simulink model "Coupled_USV_2DOF_SS_tcurve_wPID_FF_curves_2015"  (R2015b)
settings: Solver=VariableStepAuto  StartTime=0.0  StopTime=10  RelTol=1e-3
values from neighbouring files (symbols this model uses):
  breakpoints1 = data(end:-1:1,1)'    [Experimental_Impl.m]    (also in Experimental_Impl_wPlot.m; FEB02_LAKE_TEST.m; FEB14_LAKE_TEST.m; FEB28_LAKE_TEST.m)
  drag_coeff = 16.91    [Experimental_Impl.m]    (also in Experimental_Impl_wPlot.m; FEB02_LAKE_TEST.m = 8.5; FEB02_Post_Processing.m; FEB14_LAKE_TEST.m)
  Kds = .01    (= 0.01)    [FEB02_LAKE_TEST.m]    (also in FEB02_Post_Processing.m = Gain_S(3,i); FEB14_LAKE_TEST.m; FEB28_LAKE_TEST.m = 0; GainIteration_Coup.m = Gain_S(3,i))
  Kdy = Gain(3,i)    [Experimental_Impl.m]    (also in Experimental_Impl_wPlot.m; FEB02_LAKE_TEST.m = 20; FEB02_Post_Processing.m = Gain_Y(3,k); FEB14_LAKE_TEST.m = 20)
  Kis = 7    [FEB02_LAKE_TEST.m]    (also in FEB02_Post_Processing.m = Gain_S(2,i); FEB14_LAKE_TEST.m; FEB28_LAKE_TEST.m = 15; GainIteration_Coup.m = Gain_S(2,i))
  Kiy = Gain(2,i)    [Experimental_Impl.m]    (also in Experimental_Impl_wPlot.m; FEB02_LAKE_TEST.m = 0.01; FEB02_Post_Processing.m = Gain_Y(2,k); FEB14_LAKE_TEST.m = 0.01)
  Kps = 12    [FEB02_LAKE_TEST.m]    (also in FEB02_Post_Processing.m = Gain_S(1,i); FEB14_LAKE_TEST.m; FEB28_LAKE_TEST.m = 40; GainIteration_Coup.m = Gain_S(1,i))
  Kpy = Gain(1,i)    [Experimental_Impl.m]    (also in Experimental_Impl_wPlot.m; FEB02_LAKE_TEST.m = 100; FEB02_Post_Processing.m = Gain_Y(1,k); FEB14_LAKE_TEST.m = 100)
  switch_case = 0    [Experimental_Impl.m]    (also in Experimental_Impl_wPlot.m; FEB02_LAKE_TEST.m = 1; FEB02_Post_Processing.m; FEB14_LAKE_TEST.m)
  table_data = data(end:-1:1,2)'    [Experimental_Impl.m]    (also in Experimental_Impl_wPlot.m; FEB02_LAKE_TEST.m; FEB14_LAKE_TEST.m; FEB28_LAKE_TEST.m)
  vf = 0.0    (= 0)    [Experimental_Impl.m]    (also in Experimental_Impl_wPlot.m; FEB02_LAKE_TEST.m = 1.5; FEB02_Post_Processing.m = 1.25; FEB14_LAKE_TEST.m = 1.5)
  vo = 0.0    (= 0)    [Experimental_Impl.m]    (also in Experimental_Impl_wPlot.m; FEB02_LAKE_TEST.m = 1.25; FEB02_Post_Processing.m = 1.25; FEB14_LAKE_TEST.m = 1.25)
  yf = pi/4    (= 0.785398163397)    [Experimental_Impl.m]    (also in Experimental_Impl_wPlot.m = 0; FEB02_LAKE_TEST.m = 0; FEB02_Post_Processing.m = pi()/4; FEB14_LAKE_TEST.m = 0)
  yo = 0    [Experimental_Impl.m]    (also in Experimental_Impl_wPlot.m; FEB02_LAKE_TEST.m; FEB02_Post_Processing.m; FEB14_LAKE_TEST.m)
libraries: simulink_extras x1
settings Model: Creator=bsb  LastModifiedBy=aschnieders22
settings ConfigComp: CovModelRefEnable=Off

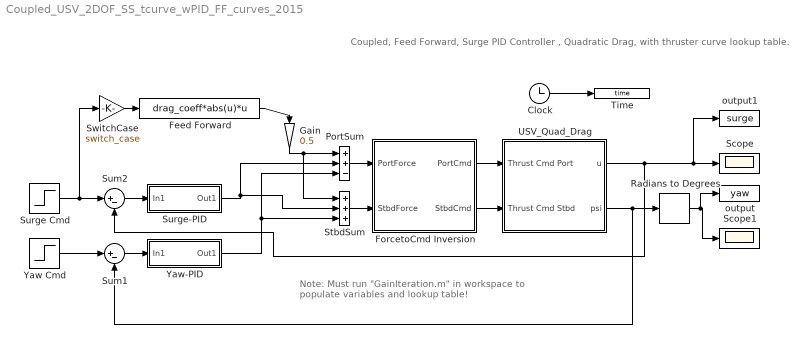
== system Coupled_USV_2DOF_SS_tcurve_wPID_FF_curves_2015 ==
  note: Note: Must run "GainIteration.m" in workspace to populate variables and lookup table!
  note: Coupled, Feed Forward, Surge PID Controller , Quadratic Drag, with thruster curve lookup table.
  Clock : Clock
  Feed Forward : Fcn  Expr=drag_coeff*abs(u)*u
  ForcetoCmd Inversion : Subsystem
  Gain : Gain  Gain=0.5
  PortSum : Sum  Inputs=++-
  Radians to Degrees : simulink_extras/Transformations/Radians to Degrees
  Scope : Scope
  Scope1 : Scope
  StbdSum : Sum  Inputs=+++
  Sum1 : Sum  Inputs=|+-
  Sum2 : Sum  Inputs=|+-
  Surge Cmd : Step  Before=vo  After=vf  SampleTime=0
  Surge-PID : Subsystem
  SwitchCase : Gain  Gain=switch_case
  Time : ToWorkspace  VariableName=time  SampleTime=-1
  USV_Quad_Drag : Subsystem
  Yaw Cmd : Step  Before=yo  After=yf  SampleTime=0
  Yaw-PID : Subsystem
  output : ToWorkspace  VariableName=yaw  SampleTime=-1
  output1 : ToWorkspace  VariableName=surge  SampleTime=-1
  wires:
  USV_Quad_Drag/2(psi) -> Sum1/2, Radians to Degrees/1
  USV_Quad_Drag/1(u) -> Sum2/2, output1/1, Scope/1
  SwitchCase/1 -> Feed Forward/1
  Clock/1 -> Time/1
  Feed Forward/1 -> Gain/1
  Gain/1 -> PortSum/1, StbdSum/1
  PortSum/1 -> ForcetoCmd Inversion/1(PortForce)
  StbdSum/1 -> ForcetoCmd Inversion/2(StbdForce)
  ForcetoCmd Inversion/1(PortCmd) -> USV_Quad_Drag/1(Thrust Cmd Port)
  ForcetoCmd Inversion/2(StbdCmd) -> USV_Quad_Drag/2(Thrust Cmd Stbd)
  Radians to Degrees/1 -> output/1, Scope1/1
  Sum1/1 -> Yaw-PID/1(In1)
  Surge Cmd/1 -> SwitchCase/1, Sum2/1
  Yaw Cmd/1 -> Sum1/1
  Yaw-PID/1(Out1) -> StbdSum/3, PortSum/3
  Sum2/1 -> Surge-PID/1(In1)
  Surge-PID/1(Out1) -> StbdSum/2, PortSum/2

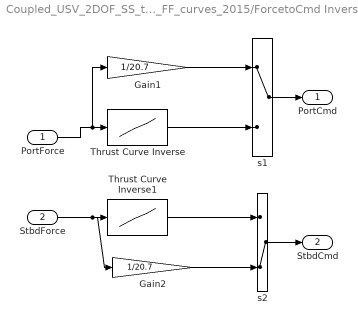
== system Coupled_USV_2DOF_SS_tcurve_wPID_FF_curves_2015/ForcetoCmd Inversion ==
  PortForce : Inport
  StbdForce : Inport  Port=2
  Gain1 : Gain  Gain=1/20.7
  Gain2 : Gain  Gain=1/20.7
  Thrust Curve Inverse : Lookup_n-D  NumberOfTableDimensions=1  BreakpointsForDimension1=table_data  Table=breakpoints1  ExtrapMethod=Clip  UseLastTableValue=on  InternalRulePriority=Speed  RndMeth=Simplest  InputSameDT=on
  Thrust Curve Inverse1 : Lookup_n-D  NumberOfTableDimensions=1  BreakpointsForDimension1=table_data  Table=breakpoints1  ExtrapMethod=Clip  UseLastTableValue=on  InternalRulePriority=Speed  RndMeth=Simplest  InputSameDT=on
  "s1 " : ManualSwitch
  s2 : ManualSwitch  CurrentSetting=0
  PortCmd : Outport
  StbdCmd : Outport  Port=2
  wires:
  StbdForce/1 -> Gain2/1, Thrust Curve Inverse1/1
  PortForce/1 -> Gain1/1, Thrust Curve Inverse/1
  Thrust Curve Inverse/1 -> "s1 "/2
  Gain1/1 -> "s1 "/1
  "s1 "/1 -> PortCmd/1
  s2/1 -> StbdCmd/1
  Thrust Curve Inverse1/1 -> s2/1
  Gain2/1 -> s2/2

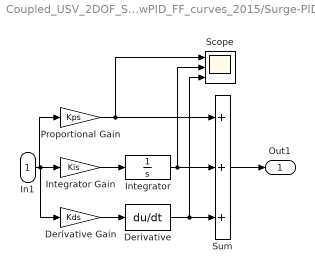
== system Coupled_USV_2DOF_SS_tcurve_wPID_FF_curves_2015/Surge-PID ==
  In1 : Inport
  Derivative : Derivative  CoefficientInTFapproximation=0
  Derivative Gain : Gain  Gain=Kds
  Integrator : TransferFcn  Denominator=[1 0]
  Integrator Gain : Gain  Gain=Kis
  Proportional Gain : Gain  Gain=Kps
  Scope : Scope  NumInputPorts=3
  Sum : Sum  Inputs=+++
  Out1 : Outport
  wires:
  Derivative Gain/1 -> Derivative/1
  Integrator Gain/1 -> Integrator/1
  Derivative/1 -> Scope/3, Sum/3
  Sum/1 -> Out1/1
  Integrator/1 -> Scope/2, Sum/2
  Proportional Gain/1 -> Scope/1, Sum/1
  In1/1 -> Derivative Gain/1, Integrator Gain/1, Proportional Gain/1

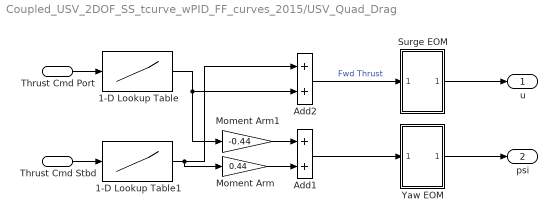
== system Coupled_USV_2DOF_SS_tcurve_wPID_FF_curves_2015/USV_Quad_Drag ==
  Thrust Cmd Port : Inport
  Thrust Cmd Stbd : Inport  Port=2
  1-D Lookup Table : Lookup_n-D  NumberOfTableDimensions=1  BreakpointsForDimension1=breakpoints1  Table=table_data  ExtrapMethod=Clip  UseLastTableValue=on  InternalRulePriority=Speed  RndMeth=Simplest  InputSameDT=on
  1-D Lookup Table1 : Lookup_n-D  NumberOfTableDimensions=1  BreakpointsForDimension1=breakpoints1  Table=table_data  ExtrapMethod=Clip  UseLastTableValue=on  InternalRulePriority=Speed  RndMeth=Simplest  InputSameDT=on
  Add1 : Sum
  Add2 : Sum
  Moment Arm : Gain  Gain=0.44
  Moment Arm1 : Gain  Gain=-0.44
  Surge EOM : Subsystem
  Yaw EOM : Subsystem
  u : Outport
  psi : Outport  Port=2
  wires:
  1-D Lookup Table/1 -> Moment Arm1/1, Add2/2
  Thrust Cmd Port/1 -> 1-D Lookup Table/1
  1-D Lookup Table1/1 -> Add2/1, Moment Arm/1
  Thrust Cmd Stbd/1 -> 1-D Lookup Table1/1
  Moment Arm1/1 -> Add1/1
  Moment Arm/1 -> Add1/2
  Add1/1 -> Yaw EOM/1(In1)
  Yaw EOM/1(Out1) -> psi/1
  Add2/1 -> Surge EOM/1(In1)  "Fwd Thrust"
  Surge EOM/1(Out1) -> u/1

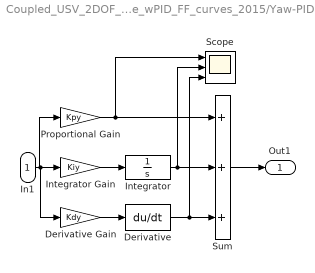
== system Coupled_USV_2DOF_SS_tcurve_wPID_FF_curves_2015/Yaw-PID ==
  In1 : Inport
  Derivative : Derivative  CoefficientInTFapproximation=0
  Derivative Gain : Gain  Gain=Kdy
  Integrator : TransferFcn  Denominator=[1 0]
  Integrator Gain : Gain  Gain=Kiy
  Proportional Gain : Gain  Gain=Kpy
  Scope : Scope  NumInputPorts=3
  Sum : Sum  Inputs=+++
  Out1 : Outport
  wires:
  Derivative Gain/1 -> Derivative/1
  Integrator Gain/1 -> Integrator/1
  Derivative/1 -> Scope/3, Sum/3
  Sum/1 -> Out1/1
  Integrator/1 -> Scope/2, Sum/2
  Proportional Gain/1 -> Scope/1, Sum/1
  In1/1 -> Derivative Gain/1, Integrator Gain/1, Proportional Gain/1

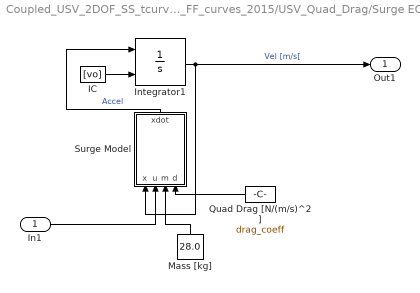
== system Coupled_USV_2DOF_SS_tcurve_wPID_FF_curves_2015/USV_Quad_Drag/Surge EOM ==
  In1 : Inport
  IC : Constant  Value=[vo]
  Integrator1 : Integrator  InitialConditionSource=external
  Mass [kg] : Constant  Value=28.0
  Quad Drag [N/(m/s)^2] : Constant  Value=drag_coeff
  Surge Model : MATLAB Function  TreatAsAtomicUnit=on
  Out1 : Outport
  wires:
  Integrator1/1 -> Out1/1, Surge Model/1(x)  "Vel [m/s["
  Surge Model/1(xdot) -> Integrator1/1  "Accel"
  In1/1 -> Surge Model/2(u)
  Mass [kg]/1 -> Surge Model/3(m)
  Quad Drag [N/(m/s)^2]/1 -> Surge Model/4(d)
  IC/1 -> Integrator1/2

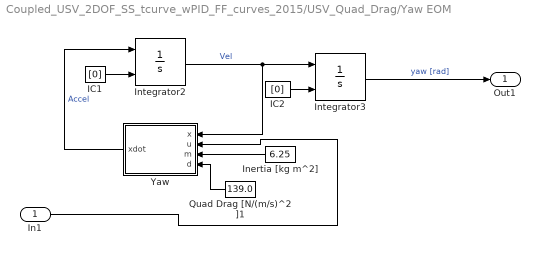
== system Coupled_USV_2DOF_SS_tcurve_wPID_FF_curves_2015/USV_Quad_Drag/Yaw EOM ==
  In1 : Inport
  IC1 : Constant  Value=[0]
  IC2 : Constant  Value=[0]
  Inertia [kg m^2] : Constant  Value=6.25
  Integrator2 : Integrator  InitialConditionSource=external
  Integrator3 : Integrator  InitialConditionSource=external
  Quad Drag [N/(m/s)^2]1 : Constant  Value=139.0
  Yaw : MATLAB Function  TreatAsAtomicUnit=on
  Out1 : Outport
  wires:
  IC1/1 -> Integrator2/2
  IC2/1 -> Integrator3/2
  In1/1 -> Yaw/2(u)
  Yaw/1(xdot) -> Integrator2/1  "Accel"
  Integrator2/1 -> Integrator3/1, Yaw/1(x)  "Vel"
  Inertia [kg m^2]/1 -> Yaw/3(m)
  Quad Drag [N/(m/s)^2]1/1 -> Yaw/4(d)
  Integrator3/1 -> Out1/1  "yaw [rad]"

== matlab function Coupled_USV_2DOF_SS_tcurve_wPID_FF_curves_2015/USV_Quad_Drag/Yaw EOM/Yaw ==
  data: x input; u input; xdot output; m input; d input
function xdot = fcn(x,u,m,d)
%#codegen

% x - state of the system.  surge velocity.
% u - input. thrust force
% Model parameters
m = m; %28.0;   % Mass [kg]
d = d; %16.9;  % Quadratic drag coefficient [N/(m/s)^2]

xdot = 1/m*(-d*abs(x)*x+u);

== matlab function Coupled_USV_2DOF_SS_tcurve_wPID_FF_curves_2015/USV_Quad_Drag/Surge EOM/Surge Model ==
  data: x input; u input; xdot output; m input; d input
function xdot = fcn(x,u,m,d)
%#codegen

% x - state of the system.  surge velocity.
% u - input. thrust force
% Model parameters
m = m; %28.0;   % Mass [kg]
d = d; %16.9;  % Quadratic drag coefficient [N/(m/s)^2]

xdot = 1/m*(-d*abs(x)*x+u);
